simulink model "Drone_Simulation"  (R2020a)
settings: Solver=ode1  StartTime=0.0  StopTime=50  FixedStep=1e-3
values from neighbouring files (symbols this model uses):
  AeEMSC = 1    [Qball_X8_Model.m]
  alpha1TDDBSC = 1    [Qball_X8_Model.m]    (also in ReliabilityModel_Script.m = 0.7)
  bBNG = 1.2    [ReliabilityModel_Script.m]
  bEMSC = 1    [Qball_X8_Model.m]
  bEVCAP = 1    [Qball_X8_Model.m]    (also in ReliabilityModel_Script.m = 1.1)
  BNG_Motor1 = 0.8    [ReliabilityModel_Script.m]
  BNG_Motor2 = 1    [ReliabilityModel_Script.m]
  BNG_Motor3 = 1    [ReliabilityModel_Script.m]
  BNG_Motor4 = 1    [ReliabilityModel_Script.m]
  BNG_Motor5 = 1    [ReliabilityModel_Script.m]
  BNG_Motor6 = 1    [ReliabilityModel_Script.m]
  bp = 0.001    [ControlLawsScript.m]    (also in ControlLaws_Script.m)
  bq = 0.001    [ControlLawsScript.m]    (also in ControlLaws_Script.m)
  br = 0.001    [ControlLawsScript.m]    (also in ControlLaws_Script.m)
  bTDDBSC = 1    [Qball_X8_Model.m]    (also in ReliabilityModel_Script.m = 1.1)
  bWDG = 1    [Qball_X8_Model.m]    (also in ReliabilityModel_Script.m = 1.1)
  C_A = [     k_T           k_T          k_T                k_T          k_T         k_T ... (first row only)    [ControlLawsScript.m]    (also in ControlLaws_Script.m)
  C_mot = 1    [Qball_X8_Model.m]    (also in ReliabilityModel_Script.m = 17.46)
  C_th_esc = 1    [Qball_X8_Model.m]    (also in ReliabilityModel_Script.m = 1.67)
  CAPEV_Motor1 = 0.8    [ReliabilityModel_Script.m]
  CAPEV_Motor2 = 1    [ReliabilityModel_Script.m]
  CAPEV_Motor3 = 1    [ReliabilityModel_Script.m]
  CAPEV_Motor4 = 1    [ReliabilityModel_Script.m]
  CAPEV_Motor5 = 1    [ReliabilityModel_Script.m]
  CAPEV_Motor6 = 1    [ReliabilityModel_Script.m]
  cdx = cx*m    (= 17.4057414746)    [ControlLawsScript.m]    (also in ControlLaws_Script.m)
  cdy = cy*m    (= 17.4057414746)    [ControlLawsScript.m]    (also in ControlLaws_Script.m)
  cdz = cz*m    (= 17.4057414746)    [ControlLawsScript.m]    (also in ControlLaws_Script.m)
  EaEMSC = 1    [Qball_X8_Model.m]
  EaEVCAP = 1    [Qball_X8_Model.m]    (also in ReliabilityModel_Script.m = 0.94)
  EalphaTDDBSC = 1    [Qball_X8_Model.m]    (also in ReliabilityModel_Script.m = 0.7)
  EaTDDBSC = 1    [Qball_X8_Model.m]    (also in ReliabilityModel_Script.m = 0.7)
  EaWDG = 1    [Qball_X8_Model.m]    (also in ReliabilityModel_Script.m = 0.5)
  g = 9.80665    [ControlLawsScript.m]    (also in ControlLaws_Script.m; Qball_X8_Model.m = 9.87)
  JrefEMSC = 1    [Qball_X8_Model.m]
  Jz = 0.15887270137511    (= 0.158872701375)    [ControlLawsScript.m]    (also in ControlLaws_Script.m)
  k_b = 1    [Qball_X8_Model.m]    (also in ReliabilityModel_Script.m = -21.8546)
  Kp = (Jx/Tc)-bp    (= 4.11390529802)    [ControlLawsScript.m]    (also in ControlLaws_Script.m)
  Kp2 = Jx*((4/ts))*((-4/ts)+((bp+Kp)/Jx))/Kp    (= 6.72163348437)    [ControlLawsScript.m]    (also in ControlLaws_Script.m)
  Kq = (Jy/Tc)-bq    (= 4.12186008142)    [ControlLawsScript.m]    (also in ControlLaws_Script.m)
  Kq2 = Jy*((4/ts))*((-4/ts)+((bq+Kq)/Jy))/Kq    (= 6.72163033191)    [ControlLawsScript.m]    (also in ControlLaws_Script.m)
  Kr = (Jz/(tsy/25))-br    (= 7.94263506876)    [ControlLawsScript.m]    (also in ControlLaws_Script.m)
  Kr2 = Jz*((4/tsy))*((-4/tsy)+((br+Kr)/Jz))/Kr    (= 6.72084606682)    [ControlLawsScript.m]    (also in ControlLaws_Script.m)
  kv = 1/930    (= 0.0010752688172)    [StingerScript.m]
  Kx = abs(Kx)    [ControlLawsScript.m]    (also in ControlLaws_Script.m)
  Ky = abs(Ky)    [ControlLawsScript.m]    (also in ControlLaws_Script.m)
  Kz = (m/Tcz)-cz    (= 38.5143536865)    [ControlLawsScript.m]    (also in ControlLaws_Script.m)
  Kz2 = m*((4/tsz))*((-4/tsz)+((cz+Kz)/m))/Kz    (= 1.89810050529)    [ControlLawsScript.m]    (also in ControlLaws_Script.m)
  LnomEMSC = 1    [Qball_X8_Model.m]
  LnomEVCAP = 1    [Qball_X8_Model.m]    (also in ReliabilityModel_Script.m = 10800000)
  LnomTDDBSC = 1    [Qball_X8_Model.m]    (also in ReliabilityModel_Script.m = 9997200)
  LnomWDG = 1    [Qball_X8_Model.m]    (also in ReliabilityModel_Script.m = 72000000)
  m = 3.4811482949175    (= 3.48114829492)    [ControlLawsScript.m]    (also in ControlLaws_Script.m; Qball_X8_Model.m = 1.45)
  max_yaw_moment = k_y*hov_thrust/k_T    (= 0.323744079512)    [ControlLawsScript.m]    (also in ControlLaws_Script.m = 0.57666914163)
  NEMSC = 1    [Qball_X8_Model.m]
  nEVCAP = 1    [Qball_X8_Model.m]    (also in ReliabilityModel_Script.m)
  pconst = 2    [Qball_X8_Model.m]    (also in ReliabilityModel_Script.m)
  pitch_angle_limit = 32/R2D    (= 0.558505360638)    [ControlLawsScript.m]    (also in ControlLaws_Script.m)
  R2D = 180/pi    (= 57.2957795131)    [ControlLawsScript.m]    (also in ControlLaws_Script.m)
  R_th_esc = 1    [Qball_X8_Model.m]    (also in ReliabilityModel_Script.m = 5.14)
  R_th_mot = 1    [Qball_X8_Model.m]    (also in ReliabilityModel_Script.m = 8.59)
  Re = 0.008    [Qball_X8_Model.m]    (also in ReliabilityModel_Script.m)
  roll_angle_limit = 32/R2D    (= 0.558505360638)    [ControlLawsScript.m]    (also in ControlLaws_Script.m)
  RrefBNG = 0.9    [ReliabilityModel_Script.m]
  RrefEMSC = 1    [Qball_X8_Model.m]
  RrefEVCAP = 1    [Qball_X8_Model.m]    (also in ReliabilityModel_Script.m = 0.9)
  RrefTDDBSC = 1    [Qball_X8_Model.m]    (also in ReliabilityModel_Script.m = 0.37)
  RrefWDG = 1    [Qball_X8_Model.m]    (also in ReliabilityModel_Script.m = 0.98)
  SCTDDB_Motor1 = 0.8    [ReliabilityModel_Script.m]
  SCTDDB_Motor2 = 1    [ReliabilityModel_Script.m]
  SCTDDB_Motor3 = 1    [ReliabilityModel_Script.m]
  SCTDDB_Motor4 = 1    [ReliabilityModel_Script.m]
  SCTDDB_Motor5 = 1    [ReliabilityModel_Script.m]
  SCTDDB_Motor6 = 1    [ReliabilityModel_Script.m]
  T_amb = 1    [Qball_X8_Model.m]    (also in ReliabilityModel_Script.m = 20)
  T_amb_mot = 1    [Qball_X8_Model.m]    (also in ReliabilityModel_Script.m = 20)
  t_D_SCTDDB = 30    [ReliabilityModel_Script.m]
  TrefEMSC = 1    [Qball_X8_Model.m]
  TrefEVCAP = 1    [Qball_X8_Model.m]    (also in ReliabilityModel_Script.m = 105)
  TrefTDDBSC = 1    [Qball_X8_Model.m]    (also in ReliabilityModel_Script.m = 150)
  TrefWDG = 1    [Qball_X8_Model.m]    (also in ReliabilityModel_Script.m = 40)
  Ub = 12    [Qball_X8_Model.m]    (also in ReliabilityModel_Script.m)
  VmaxEVCAP = 1    [Qball_X8_Model.m]    (also in ReliabilityModel_Script.m = 35)
  VnomEVCAP = 1    [Qball_X8_Model.m]    (also in ReliabilityModel_Script.m = 35)
  WDG_Motor1 = 0.8    [ReliabilityModel_Script.m]
  WDG_Motor2 = 1    [ReliabilityModel_Script.m]
  WDG_Motor3 = 1    [ReliabilityModel_Script.m]
  WDG_Motor4 = 1    [ReliabilityModel_Script.m]
  WDG_Motor5 = 1    [ReliabilityModel_Script.m]
  WDG_Motor6 = 1    [ReliabilityModel_Script.m]
  z_x = cx    (= 5)    [ControlLawsScript.m]    (also in ControlLaws_Script.m)
  z_y = cy    (= 5)    [ControlLawsScript.m]    (also in ControlLaws_Script.m)
undefined symbols (not defined in the file or in its folder): FuselageContactForces, LeftAftArm, LeftAftSkid, LeftArm, LeftFrontArm, LeftFrontSkid, LeftSideContactForces, Lower, missionPlanX, missionPlanY, missionPlanYaw, missionPlanZ, Newton, Raphson, RightAftArm, RightAftSkid, RightArm, RightFrontArm, RightFrontSkid, RightSideContactForces, SkidsContactForces, timeConstant, Upper, X, Y, Z
libraries: sm_lib x90, nesl_utility x78, fl_lib x61, ee_lib x19, dspinverses x1, dspmtrx3 x1
(part 4 of 5)

== system Drone_Simulation/PLANT MODEL/ELECTRIC SYSTEM/Motor 4 ==
  Aerodynamic Drag : fl_lib/Mechanical/Mechanical Sources/Ideal Torque Source
  Controlled PWM Voltage : ee_lib/Integrated Circuits/Controlled PWM Voltage  F=freq Hz  TD=0 s  pulse_width_offset=0 s  pulse_min=0 s  Vmin=0 V  Vmax=5 V  Vm=1 V  pwm_or_av=1  event_type=2  sample_time=Samp_time s  u_min=0  u_max=1
      settings: InternalSimscapePortConfiguration="{\"Bottom\":[],\"Left\":[{\"id\":\"u\",\"label\":\"u\",\"type\":\"input\"}],\"Right\":[{\"id\":\"p2\",\"label\":\"PWM\",\"type\":\"foundation.electrical.electrical\"},{\"id\":\"n2\",\"label\":\"REF\",\"type\":\"foundation.electrical.electrical\"}],\"Top\":[]}"
  Current Sensor : fl_lib/Electrical/Electrical Sensors/Current Sensor
  DC Motor : ee_lib/Electromechanical/Brushed Motors/DC Motor  field_option=ee.enum.field_option.pm  Rf=100 Ohm  Lf=1 H  Laf=0.15 H  If0=0 A  parameterization=ee.enum.dcparam_option.circuit_param  Ra=R Ohm  La=100 uH  emf_or_torque=ee.enum.emf_or_torque.kv  Kv=Kv V/rpm  Ki=kv N*m/A  T_stall=0.1 N*m  w_max=4000 rpm  w_rated=2500 rpm  P_rated=10 W  V_rated=12 V  J=0 kg*m^2  lam_param=ee.enum.lam_param.current  lam=0.5e-5 N*m/(rad/s)  i_noload=Ic A  V_i_noload=14.8 V  speed0=0 rpm  alpha=3.93e-3 1/K  Tmeas=25 degC  thermal_mass=100 J/K  initial_temperature=25 degC
  H-Bridge : ee_lib/Semiconductors & Converters/Converters/H-Bridge  supply_ports=ee.enum.supply_ports.showsupply  Venable=0.01 V  Vmax=5 V  Vreverse=10000 V  Vbrake=10000 V  Vm=12 V  pwm_or_av=ee.enum.pwm_or_av.pwm  regenerative_braking_mode=ee.enum.converters.regenerative_braking_mode.always_enabled  discontinuous=ee.enum.current_profile.continuous  freewheeling_mode=ee.enum.converters.freewheeling_mode.two_switches_one_diode  Ron=0.00001 Ohm  Don=0.1 Ohm  Goff=1e-6 S  Rload=3.38+0.1 Ohm  Lload=1e-5 H  F=4 kHz  thermal_mass=100 J/K  initial_temperature=298.15 K  Ron2=0.1 Ohm  Don2=0.05 Ohm  Tmeas=298.15 K  Tmeas2=398.15 K
      settings: InternalSimscapePortConfiguration="{\"Bottom\":[],\"Left\":[{\"id\":\"ENA\",\"label\":\"PWM\",\"type\":\"foundation.electrical.electrical\"},{\"id\":\"REF\",\"label\":\"REF\",\"type\":\"foundation.electrical.electrical\"},{\"id\":\"REV\",\"label\":\"REV\",\"type\":\"foundation.electrical.electrical\"},{\"id\":\"BRK\",\"label\":\"BRK\",\"type\":\"foundation.electrical.electrical\"}],\"Right\":[{\"id\":\"p1\",\"label\":\"V+\",\"type\":\"foundation.electrical.electrical\"},{\"id\":\"p2\",\"label\":\"+\",\"type\":\"foundation.electrical.electrical\"},{\"id\":\"n2\",\"label\":\"-\",\"type\":\"foundation.electrical.electrical\"},{\"id\":\"n1\",\"label\":\"V-\",\"type\":\"foundation.electrical.electrical\"}],\"Top\":[]}"
  Ideal Rotational Motion Sensor : fl_lib/Mechanical/Mechanical Sensors/Ideal Rotational Motion Sensor  wrap_angle=simscape.enum.onoff.off  offset=0 deg
  Ideal Torque Sensor : fl_lib/Mechanical/Mechanical Sensors/Ideal Torque Sensor
  MRRef : fl_lib/Mechanical/Rotational Elements/Mechanical Rotational Reference
  Mechanical Rotational Reference2 : fl_lib/Mechanical/Rotational Elements/Mechanical Rotational Reference
  PS-Simulink : nesl_utility/PS-Simulink Converter  PhysicalDomain=network_engine_domain  SubClassName=ps_output  LeftPortType=input  RightPortType=output  PseudoPeriodic=off  Frequencies=[]  Unit=rpm  AffineConversion=off
  PS-Simulink Converter : nesl_utility/PS-Simulink Converter  PhysicalDomain=network_engine_domain  SubClassName=ps_output  LeftPortType=input  RightPortType=output  PseudoPeriodic=off  Frequencies=[]  Unit=inherit  AffineConversion=off
  PS-Simulink Converter1 : nesl_utility/PS-Simulink Converter  PhysicalDomain=network_engine_domain  SubClassName=ps_output  LeftPortType=input  RightPortType=output  PseudoPeriodic=off  Frequencies=[]  Unit=inherit  AffineConversion=off
  PS-Simulink Converter3 : nesl_utility/PS-Simulink Converter  PhysicalDomain=network_engine_domain  SubClassName=ps_output  LeftPortType=input  RightPortType=output  PseudoPeriodic=off  Frequencies=[]  Unit=inherit  AffineConversion=off
  PS-Simulink3 : nesl_utility/PS-Simulink Converter  PhysicalDomain=network_engine_domain  SubClassName=ps_output  LeftPortType=input  RightPortType=output  PseudoPeriodic=off  Frequencies=[]  Unit=A  AffineConversion=off
  Propeller Inertia : fl_lib/Mechanical/Rotational Elements/Inertia  inertia=J kg*m^2  w_specify=off  w_priority=High  w=0 rpm  w_nominal_specify=off  w_nominal_unit=rad/s  w_nominal_value=1  t_specify=off  t_priority=High  t=0 N*m  t_nominal_specify=off  t_nominal_unit=N*m  t_nominal_value=1
  RPM to Resistive Torque and Thrust : Subsystem
  Scope2 : Scope
  Signals : Subsystem
  Simulink-PS Converter : nesl_utility/Simulink-PS Converter  PhysicalDomain=network_engine_domain  SubClassName=ps_input  LeftPortType=input  RightPortType=output  PseudoPeriodic=off  Frequencies=[]  NoiseDistribution=none  NoiseParameters=[]  Unit=1  AffineConversion=off  FilteringAndDerivatives=filter  SimscapeFilterOrder=1  InputFilterTimeConstant=0.001  UdotUserProvided=0
  Simulink-PS Converter1 : nesl_utility/Simulink-PS Converter  PhysicalDomain=network_engine_domain  SubClassName=ps_input  LeftPortType=input  RightPortType=output  PseudoPeriodic=off  Frequencies=[]  NoiseDistribution=none  NoiseParameters=[]  Unit=N*m  AffineConversion=off  FilteringAndDerivatives=provide  SimscapeFilterOrder=1  InputFilterTimeConstant=0.001  UdotUserProvided=0
  Sum : Sum  Inputs=|+-
  Terminator : Terminator
  Transfer Fcn2 : TransferFcn  Numerator=[1*2*pi]  Denominator=[1 1*2*pi]
  Transfer Fcn3 : TransferFcn  Numerator=[1*2*pi]  Denominator=[1 1*2*pi]
  Visualization : Scope  NumInputPorts=4
  Voltage Sensor1 : fl_lib/Electrical/Electrical Sensors/Voltage Sensor
  Connection Port1 : PMIOPort  Side=Left
  Connection Port : PMIOPort  Port=2  Side=Right
  tag scope: AngleMotor4=global, AngularSpeed4=global, I_ESC_OUT4=global, Thrust4=global, Trq4=global, V_ESC_OUT4=global
  wires:
  RPM to Resistive Torque and Thrust/2(Resistive Torque) -> [Trq4], Simulink-PS Converter1/1  "Torque"
  [AngularSpeed4] -> RPM to Resistive Torque and Thrust/1(Angular Speed)
  RPM to Resistive Torque and Thrust/1(Thrust) -> [Thrust4]  "Thrust"
  PS-Simulink Converter1/1 -> Terminator/1
  PS-Simulink/1 -> Scope2/1, Sum/2, [AngularSpeed4]  "Motor RPM"
  [ReqSpeedMotor4] -> Sum/1  "Motor Desired Speed"
  Transfer Fcn2/1 -> [I_ESC_OUT4]
  PS-Simulink3/1 -> Transfer Fcn2/1  "Motor Current"
  PS-Simulink Converter3/1 -> Transfer Fcn3/1  "Motor Voltage"
  Transfer Fcn3/1 -> [V_ESC_OUT4]
  PS-Simulink Converter/1 -> [AngleMotor4]
  Sum/1 -> Simulink-PS Converter/1
  Signals/4(V) -> Visualization/4
  Signals/3(Trq) -> Visualization/3
  Signals/2(ia) -> Visualization/2
  Signals/1(Spd) -> Visualization/1
  connections:
  Ideal Rotational Motion Sensor/RConn2 -- PS-Simulink/LConn1
  PS-Simulink Converter1/LConn1 -- Ideal Torque Sensor/RConn2
  Ideal Torque Sensor/RConn1 -- Aerodynamic Drag/LConn1
  Simulink-PS Converter1/RConn1 -- Aerodynamic Drag/RConn1
  Mechanical Rotational Reference2/LConn1 -- Aerodynamic Drag/RConn2
  Ideal Torque Sensor/LConn1 -- DC Motor/LConn2 -- Propeller Inertia/LConn1 -- Ideal Rotational Motion Sensor/LConn1
  Ideal Rotational Motion Sensor/RConn1 -- MRRef/LConn1 -- DC Motor/RConn2
  H-Bridge/RConn4 -- Connection Port/RConn1 -- H-Bridge/LConn3 -- Controlled PWM Voltage/RConn2 -- H-Bridge/LConn2 -- H-Bridge/LConn4
  Controlled PWM Voltage/RConn1 -- H-Bridge/LConn1
  Simulink-PS Converter/RConn1 -- Controlled PWM Voltage/LConn1
  H-Bridge/RConn3 -- Voltage Sensor1/RConn2 -- DC Motor/RConn1
  Connection Port1/RConn1 -- H-Bridge/RConn1
  Current Sensor/LConn1 -- Voltage Sensor1/LConn1 -- H-Bridge/RConn2
  PS-Simulink3/LConn1 -- Current Sensor/RConn1
  Current Sensor/RConn2 -- DC Motor/LConn1
  Voltage Sensor1/RConn1 -- PS-Simulink Converter3/LConn1
  PS-Simulink Converter/LConn1 -- Ideal Rotational Motion Sensor/RConn3

== system Drone_Simulation/PLANT MODEL/ELECTRIC SYSTEM/Motor 5 ==
  Aerodynamic Drag : fl_lib/Mechanical/Mechanical Sources/Ideal Torque Source
  Controlled PWM Voltage : ee_lib/Integrated Circuits/Controlled PWM Voltage  F=freq Hz  TD=0 s  pulse_width_offset=0 s  pulse_min=0 s  Vmin=0 V  Vmax=5 V  Vm=1 V  pwm_or_av=1  event_type=2  sample_time=Samp_time s  u_min=0  u_max=1
      settings: InternalSimscapePortConfiguration="{\"Bottom\":[],\"Left\":[{\"id\":\"u\",\"label\":\"u\",\"type\":\"input\"}],\"Right\":[{\"id\":\"p2\",\"label\":\"PWM\",\"type\":\"foundation.electrical.electrical\"},{\"id\":\"n2\",\"label\":\"REF\",\"type\":\"foundation.electrical.electrical\"}],\"Top\":[]}"
  Current Sensor : fl_lib/Electrical/Electrical Sensors/Current Sensor
  DC Motor : ee_lib/Electromechanical/Brushed Motors/DC Motor  field_option=ee.enum.field_option.pm  Rf=100 Ohm  Lf=1 H  Laf=0.15 H  If0=0 A  parameterization=ee.enum.dcparam_option.circuit_param  Ra=R Ohm  La=100 uH  emf_or_torque=ee.enum.emf_or_torque.kv  Kv=Kv V/rpm  Ki=kv N*m/A  T_stall=0.1 N*m  w_max=4000 rpm  w_rated=2500 rpm  P_rated=10 W  V_rated=12 V  J=0 kg*m^2  lam_param=ee.enum.lam_param.current  lam=0.5e-5 N*m/(rad/s)  i_noload=Ic A  V_i_noload=14.8 V  speed0=0 rpm  alpha=3.93e-3 1/K  Tmeas=25 degC  thermal_mass=100 J/K  initial_temperature=25 degC
  H-Bridge : ee_lib/Semiconductors & Converters/Converters/H-Bridge  supply_ports=ee.enum.supply_ports.showsupply  Venable=0.01 V  Vmax=5 V  Vreverse=10000 V  Vbrake=10000 V  Vm=12 V  pwm_or_av=ee.enum.pwm_or_av.pwm  regenerative_braking_mode=ee.enum.converters.regenerative_braking_mode.always_enabled  discontinuous=ee.enum.current_profile.continuous  freewheeling_mode=ee.enum.converters.freewheeling_mode.two_switches_one_diode  Ron=0.00001 Ohm  Don=0.1 Ohm  Goff=1e-6 S  Rload=3.38+0.1 Ohm  Lload=1e-5 H  F=4 kHz  thermal_mass=100 J/K  initial_temperature=298.15 K  Ron2=0.1 Ohm  Don2=0.05 Ohm  Tmeas=298.15 K  Tmeas2=398.15 K
      settings: InternalSimscapePortConfiguration="{\"Bottom\":[],\"Left\":[{\"id\":\"ENA\",\"label\":\"PWM\",\"type\":\"foundation.electrical.electrical\"},{\"id\":\"REF\",\"label\":\"REF\",\"type\":\"foundation.electrical.electrical\"},{\"id\":\"REV\",\"label\":\"REV\",\"type\":\"foundation.electrical.electrical\"},{\"id\":\"BRK\",\"label\":\"BRK\",\"type\":\"foundation.electrical.electrical\"}],\"Right\":[{\"id\":\"p1\",\"label\":\"V+\",\"type\":\"foundation.electrical.electrical\"},{\"id\":\"p2\",\"label\":\"+\",\"type\":\"foundation.electrical.electrical\"},{\"id\":\"n2\",\"label\":\"-\",\"type\":\"foundation.electrical.electrical\"},{\"id\":\"n1\",\"label\":\"V-\",\"type\":\"foundation.electrical.electrical\"}],\"Top\":[]}"
  Ideal Rotational Motion Sensor : fl_lib/Mechanical/Mechanical Sensors/Ideal Rotational Motion Sensor  wrap_angle=simscape.enum.onoff.off  offset=0 deg
  Ideal Torque Sensor : fl_lib/Mechanical/Mechanical Sensors/Ideal Torque Sensor
  MRRef : fl_lib/Mechanical/Rotational Elements/Mechanical Rotational Reference
  Mechanical Rotational Reference2 : fl_lib/Mechanical/Rotational Elements/Mechanical Rotational Reference
  PS-Simulink : nesl_utility/PS-Simulink Converter  PhysicalDomain=network_engine_domain  SubClassName=ps_output  LeftPortType=input  RightPortType=output  PseudoPeriodic=off  Frequencies=[]  Unit=rpm  AffineConversion=off
  PS-Simulink Converter : nesl_utility/PS-Simulink Converter  PhysicalDomain=network_engine_domain  SubClassName=ps_output  LeftPortType=input  RightPortType=output  PseudoPeriodic=off  Frequencies=[]  Unit=inherit  AffineConversion=off
  PS-Simulink Converter1 : nesl_utility/PS-Simulink Converter  PhysicalDomain=network_engine_domain  SubClassName=ps_output  LeftPortType=input  RightPortType=output  PseudoPeriodic=off  Frequencies=[]  Unit=inherit  AffineConversion=off
  PS-Simulink Converter3 : nesl_utility/PS-Simulink Converter  PhysicalDomain=network_engine_domain  SubClassName=ps_output  LeftPortType=input  RightPortType=output  PseudoPeriodic=off  Frequencies=[]  Unit=inherit  AffineConversion=off
  PS-Simulink3 : nesl_utility/PS-Simulink Converter  PhysicalDomain=network_engine_domain  SubClassName=ps_output  LeftPortType=input  RightPortType=output  PseudoPeriodic=off  Frequencies=[]  Unit=A  AffineConversion=off
  Propeller Inertia : fl_lib/Mechanical/Rotational Elements/Inertia  inertia=J kg*m^2  w_specify=off  w_priority=High  w=0 rpm  w_nominal_specify=off  w_nominal_unit=rad/s  w_nominal_value=1  t_specify=off  t_priority=High  t=0 N*m  t_nominal_specify=off  t_nominal_unit=N*m  t_nominal_value=1
  RPM to Resistive Torque and Thrust : Subsystem
  Scope3 : Scope
  Signals : Subsystem
  Simulink-PS Converter : nesl_utility/Simulink-PS Converter  PhysicalDomain=network_engine_domain  SubClassName=ps_input  LeftPortType=input  RightPortType=output  PseudoPeriodic=off  Frequencies=[]  NoiseDistribution=none  NoiseParameters=[]  Unit=1  AffineConversion=off  FilteringAndDerivatives=filter  SimscapeFilterOrder=1  InputFilterTimeConstant=0.001  UdotUserProvided=0
  Simulink-PS Converter1 : nesl_utility/Simulink-PS Converter  PhysicalDomain=network_engine_domain  SubClassName=ps_input  LeftPortType=input  RightPortType=output  PseudoPeriodic=off  Frequencies=[]  NoiseDistribution=none  NoiseParameters=[]  Unit=N*m  AffineConversion=off  FilteringAndDerivatives=provide  SimscapeFilterOrder=1  InputFilterTimeConstant=0.001  UdotUserProvided=0
  Sum : Sum  Inputs=|+-
  Terminator : Terminator
  Transfer Fcn2 : TransferFcn  Numerator=[1*2*pi]  Denominator=[1 1*2*pi]
  Transfer Fcn3 : TransferFcn  Numerator=[1*2*pi]  Denominator=[1 1*2*pi]
  Visualization : Scope  NumInputPorts=4
  Voltage Sensor1 : fl_lib/Electrical/Electrical Sensors/Voltage Sensor
  Connection Port1 : PMIOPort  Side=Left
  Connection Port : PMIOPort  Port=2  Side=Right
  tag scope: AngleMotor5=global, AngularSpeed5=global, I_ESC_OUT5=global, Thrust5=global, Trq5=global, V_ESC_OUT5=global
  wires:
  RPM to Resistive Torque and Thrust/2(Resistive Torque) -> [Trq5], Simulink-PS Converter1/1  "Torque"
  [AngularSpeed5] -> RPM to Resistive Torque and Thrust/1(Angular Speed)
  RPM to Resistive Torque and Thrust/1(Thrust) -> [Thrust5]  "Thrust"
  PS-Simulink Converter1/1 -> Terminator/1
  PS-Simulink/1 -> Scope3/1, Sum/2, [AngularSpeed5]  "Motor RPM"
  [ReqSpeedMotor5] -> Sum/1  "Motor Desired Speed"
  PS-Simulink3/1 -> Transfer Fcn2/1  "Motor Current"
  Transfer Fcn2/1 -> [I_ESC_OUT5]
  PS-Simulink Converter3/1 -> Transfer Fcn3/1  "Motor Voltage"
  Transfer Fcn3/1 -> [V_ESC_OUT5]
  PS-Simulink Converter/1 -> [AngleMotor5]
  Sum/1 -> Simulink-PS Converter/1
  Signals/4(V) -> Visualization/4
  Signals/3(Trq) -> Visualization/3
  Signals/2(ia) -> Visualization/2
  Signals/1(Spd) -> Visualization/1
  connections:
  Ideal Rotational Motion Sensor/RConn2 -- PS-Simulink/LConn1
  PS-Simulink Converter1/LConn1 -- Ideal Torque Sensor/RConn2
  Ideal Torque Sensor/RConn1 -- Aerodynamic Drag/LConn1
  Simulink-PS Converter1/RConn1 -- Aerodynamic Drag/RConn1
  Mechanical Rotational Reference2/LConn1 -- Aerodynamic Drag/RConn2
  Ideal Torque Sensor/LConn1 -- DC Motor/LConn2 -- Propeller Inertia/LConn1 -- Ideal Rotational Motion Sensor/LConn1
  Ideal Rotational Motion Sensor/RConn1 -- MRRef/LConn1 -- DC Motor/RConn2
  Connection Port/RConn1 -- H-Bridge/RConn4 -- H-Bridge/LConn3 -- Controlled PWM Voltage/RConn2 -- H-Bridge/LConn2 -- H-Bridge/LConn4
  H-Bridge/RConn2 -- Voltage Sensor1/LConn1 -- Current Sensor/LConn1
  Controlled PWM Voltage/RConn1 -- H-Bridge/LConn1
  Simulink-PS Converter/RConn1 -- Controlled PWM Voltage/LConn1
  H-Bridge/RConn3 -- DC Motor/RConn1 -- Voltage Sensor1/RConn2
  Connection Port1/RConn1 -- H-Bridge/RConn1
  PS-Simulink3/LConn1 -- Current Sensor/RConn1
  Current Sensor/RConn2 -- DC Motor/LConn1
  Voltage Sensor1/RConn1 -- PS-Simulink Converter3/LConn1
  PS-Simulink Converter/LConn1 -- Ideal Rotational Motion Sensor/RConn3

== system Drone_Simulation/PLANT MODEL/ELECTRIC SYSTEM/Motor 6 ==
  Aerodynamic Drag : fl_lib/Mechanical/Mechanical Sources/Ideal Torque Source
  Controlled PWM Voltage : ee_lib/Integrated Circuits/Controlled PWM Voltage  F=freq Hz  TD=0 s  pulse_width_offset=0 s  pulse_min=0 s  Vmin=0 V  Vmax=5 V  Vm=1 V  pwm_or_av=1  event_type=2  sample_time=Samp_time s  u_min=0  u_max=1
      settings: InternalSimscapePortConfiguration="{\"Bottom\":[],\"Left\":[{\"id\":\"u\",\"label\":\"u\",\"type\":\"input\"}],\"Right\":[{\"id\":\"p2\",\"label\":\"PWM\",\"type\":\"foundation.electrical.electrical\"},{\"id\":\"n2\",\"label\":\"REF\",\"type\":\"foundation.electrical.electrical\"}],\"Top\":[]}"
  Current Sensor : fl_lib/Electrical/Electrical Sensors/Current Sensor
  DC Motor : ee_lib/Electromechanical/Brushed Motors/DC Motor  field_option=ee.enum.field_option.pm  Rf=100 Ohm  Lf=1 H  Laf=0.15 H  If0=0 A  parameterization=ee.enum.dcparam_option.circuit_param  Ra=R Ohm  La=100 uH  emf_or_torque=ee.enum.emf_or_torque.kv  Kv=Kv V/rpm  Ki=kv N*m/A  T_stall=0.1 N*m  w_max=4000 rpm  w_rated=2500 rpm  P_rated=10 W  V_rated=12 V  J=0 kg*m^2  lam_param=ee.enum.lam_param.current  lam=0.5e-5 N*m/(rad/s)  i_noload=Ic A  V_i_noload=14.8 V  speed0=0 rpm  alpha=3.93e-3 1/K  Tmeas=25 degC  thermal_mass=100 J/K  initial_temperature=25 degC
  H-Bridge : ee_lib/Semiconductors & Converters/Converters/H-Bridge  supply_ports=ee.enum.supply_ports.showsupply  Venable=0.01 V  Vmax=5 V  Vreverse=10000 V  Vbrake=10000 V  Vm=12 V  pwm_or_av=ee.enum.pwm_or_av.pwm  regenerative_braking_mode=ee.enum.converters.regenerative_braking_mode.always_enabled  discontinuous=ee.enum.current_profile.continuous  freewheeling_mode=ee.enum.converters.freewheeling_mode.two_switches_one_diode  Ron=0.00001 Ohm  Don=0.1 Ohm  Goff=1e-6 S  Rload=3.38+0.1 Ohm  Lload=1e-5 H  F=4 kHz  thermal_mass=100 J/K  initial_temperature=298.15 K  Ron2=0.1 Ohm  Don2=0.05 Ohm  Tmeas=298.15 K  Tmeas2=398.15 K
      settings: InternalSimscapePortConfiguration="{\"Bottom\":[],\"Left\":[{\"id\":\"ENA\",\"label\":\"PWM\",\"type\":\"foundation.electrical.electrical\"},{\"id\":\"REF\",\"label\":\"REF\",\"type\":\"foundation.electrical.electrical\"},{\"id\":\"REV\",\"label\":\"REV\",\"type\":\"foundation.electrical.electrical\"},{\"id\":\"BRK\",\"label\":\"BRK\",\"type\":\"foundation.electrical.electrical\"}],\"Right\":[{\"id\":\"p1\",\"label\":\"V+\",\"type\":\"foundation.electrical.electrical\"},{\"id\":\"p2\",\"label\":\"+\",\"type\":\"foundation.electrical.electrical\"},{\"id\":\"n2\",\"label\":\"-\",\"type\":\"foundation.electrical.electrical\"},{\"id\":\"n1\",\"label\":\"V-\",\"type\":\"foundation.electrical.electrical\"}],\"Top\":[]}"
  Ideal Rotational Motion Sensor : fl_lib/Mechanical/Mechanical Sensors/Ideal Rotational Motion Sensor  wrap_angle=simscape.enum.onoff.off  offset=0 deg
  Ideal Torque Sensor : fl_lib/Mechanical/Mechanical Sensors/Ideal Torque Sensor
  MRRef : fl_lib/Mechanical/Rotational Elements/Mechanical Rotational Reference
  Mechanical Rotational Reference2 : fl_lib/Mechanical/Rotational Elements/Mechanical Rotational Reference
  PS-Simulink : nesl_utility/PS-Simulink Converter  PhysicalDomain=network_engine_domain  SubClassName=ps_output  LeftPortType=input  RightPortType=output  PseudoPeriodic=off  Frequencies=[]  Unit=rpm  AffineConversion=off
  PS-Simulink Converter : nesl_utility/PS-Simulink Converter  PhysicalDomain=network_engine_domain  SubClassName=ps_output  LeftPortType=input  RightPortType=output  PseudoPeriodic=off  Frequencies=[]  Unit=inherit  AffineConversion=off
  PS-Simulink Converter1 : nesl_utility/PS-Simulink Converter  PhysicalDomain=network_engine_domain  SubClassName=ps_output  LeftPortType=input  RightPortType=output  PseudoPeriodic=off  Frequencies=[]  Unit=inherit  AffineConversion=off
  PS-Simulink Converter3 : nesl_utility/PS-Simulink Converter  PhysicalDomain=network_engine_domain  SubClassName=ps_output  LeftPortType=input  RightPortType=output  PseudoPeriodic=off  Frequencies=[]  Unit=inherit  AffineConversion=off
  PS-Simulink3 : nesl_utility/PS-Simulink Converter  PhysicalDomain=network_engine_domain  SubClassName=ps_output  LeftPortType=input  RightPortType=output  PseudoPeriodic=off  Frequencies=[]  Unit=A  AffineConversion=off
  Propeller Inertia : fl_lib/Mechanical/Rotational Elements/Inertia  inertia=J kg*m^2  w_specify=off  w_priority=High  w=0 rpm  w_nominal_specify=off  w_nominal_unit=rad/s  w_nominal_value=1  t_specify=off  t_priority=High  t=0 N*m  t_nominal_specify=off  t_nominal_unit=N*m  t_nominal_value=1
  RPM to Resistive Torque and Thrust : Subsystem
  Signals : Subsystem
  Simulink-PS Converter : nesl_utility/Simulink-PS Converter  PhysicalDomain=network_engine_domain  SubClassName=ps_input  LeftPortType=input  RightPortType=output  PseudoPeriodic=off  Frequencies=[]  NoiseDistribution=none  NoiseParameters=[]  Unit=1  AffineConversion=off  FilteringAndDerivatives=filter  SimscapeFilterOrder=1  InputFilterTimeConstant=0.001  UdotUserProvided=0
  Simulink-PS Converter1 : nesl_utility/Simulink-PS Converter  PhysicalDomain=network_engine_domain  SubClassName=ps_input  LeftPortType=input  RightPortType=output  PseudoPeriodic=off  Frequencies=[]  NoiseDistribution=none  NoiseParameters=[]  Unit=N*m  AffineConversion=off  FilteringAndDerivatives=provide  SimscapeFilterOrder=1  InputFilterTimeConstant=0.001  UdotUserProvided=0
  Sum : Sum  Inputs=|+-
  Terminator : Terminator
  Transfer Fcn2 : TransferFcn  Numerator=[1*2*pi]  Denominator=[1 1*2*pi]
  Transfer Fcn3 : TransferFcn  Numerator=[1*2*pi]  Denominator=[1 1*2*pi]
  Visualization : Scope  NumInputPorts=4
  Voltage Sensor1 : fl_lib/Electrical/Electrical Sensors/Voltage Sensor
  Connection Port1 : PMIOPort  Side=Left
  Connection Port : PMIOPort  Port=2  Side=Right
  tag scope: AngleMotor6=global, AngularSpeed6=global, I_ESC_OUT6=global, Thrust6=global, Trq6=global, V_ESC_OUT6=global
  wires:
  RPM to Resistive Torque and Thrust/2(Resistive Torque) -> [Trq6], Simulink-PS Converter1/1  "Torque"
  [AngularSpeed6] -> RPM to Resistive Torque and Thrust/1(Angular Speed)
  RPM to Resistive Torque and Thrust/1(Thrust) -> [Thrust6]  "Thrust"
  PS-Simulink Converter1/1 -> Terminator/1
  PS-Simulink/1 -> Sum/2, [AngularSpeed6]  "Motor RPM"
  [ReqSpeedMotor6] -> Sum/1  "Motor Desired Speed"
  PS-Simulink3/1 -> Transfer Fcn2/1  "Motor Current"
  Transfer Fcn2/1 -> [I_ESC_OUT6]
  Transfer Fcn3/1 -> [V_ESC_OUT6]
  PS-Simulink Converter3/1 -> Transfer Fcn3/1  "Motor Voltage"
  PS-Simulink Converter/1 -> [AngleMotor6]
  Sum/1 -> Simulink-PS Converter/1
  Signals/3(Trq) -> Visualization/3
  Signals/1(Spd) -> Visualization/1
  Signals/4(V) -> Visualization/4
  Signals/2(ia) -> Visualization/2
  connections:
  Ideal Rotational Motion Sensor/RConn2 -- PS-Simulink/LConn1
  PS-Simulink Converter1/LConn1 -- Ideal Torque Sensor/RConn2
  Ideal Torque Sensor/RConn1 -- Aerodynamic Drag/LConn1
  Simulink-PS Converter1/RConn1 -- Aerodynamic Drag/RConn1
  Mechanical Rotational Reference2/LConn1 -- Aerodynamic Drag/RConn2
  Ideal Torque Sensor/LConn1 -- DC Motor/LConn2 -- Propeller Inertia/LConn1 -- Ideal Rotational Motion Sensor/LConn1
  Ideal Rotational Motion Sensor/RConn1 -- MRRef/LConn1 -- DC Motor/RConn2
  H-Bridge/RConn4 -- H-Bridge/LConn3 -- Controlled PWM Voltage/RConn2 -- H-Bridge/LConn2 -- H-Bridge/LConn4 -- Connection Port/RConn1
  H-Bridge/RConn2 -- Voltage Sensor1/LConn1 -- Current Sensor/LConn1
  Controlled PWM Voltage/RConn1 -- H-Bridge/LConn1
  Controlled PWM Voltage/LConn1 -- Simulink-PS Converter/RConn1
  DC Motor/RConn1 -- H-Bridge/RConn3 -- Voltage Sensor1/RConn2
  Connection Port1/RConn1 -- H-Bridge/RConn1
  PS-Simulink3/LConn1 -- Current Sensor/RConn1
  Current Sensor/RConn2 -- DC Motor/LConn1
  Voltage Sensor1/RConn1 -- PS-Simulink Converter3/LConn1
  PS-Simulink Converter/LConn1 -- Ideal Rotational Motion Sensor/RConn3

== system Drone_Simulation/PLANT MODEL/ELECTRIC SYSTEM/Subsystem ==
  In1 : Inport
  1-D Lookup Table : Lookup_n-D  NumberOfTableDimensions=1  BreakpointsForDimension1=[0,0.05,0.1,0.15,0.2,0.25,0.3,0.35,0.4,0.45,0.5,0.55,0.6,0.65,0.7,0.75,0.8,0.85,0.9,0.95,1]  Table=[0,12,13,13.4,13.62,13.75,13.85,13.91,13.95,14,14,14,14,14,14,14,14,14,14,14.8,16.8]  InternalRulePriority=Speed  RndMeth=Simplest  InputSameDT=on
  Battery Capacity : Constant  Value=18720
  Current Sign Saturation : Saturate  UpperLimit=350  LowerLimit=0
  Current integration : Integrator
  SOC Fraction : Product  Inputs=/*
  Scope1 : Scope
  Simulink-PS Converter : nesl_utility/Simulink-PS Converter  PhysicalDomain=network_engine_domain  SubClassName=ps_input  LeftPortType=input  RightPortType=output  PseudoPeriodic=off  Frequencies=[]  NoiseDistribution=none  NoiseParameters=[]  Unit=V  AffineConversion=off  FilteringAndDerivatives=filter  SimscapeFilterOrder=1  InputFilterTimeConstant=0.001  UdotUserProvided=0
  Sum : Sum  Inputs=+|-
  output : PMIOPort  Side=Right
  wires:
  Battery Capacity/1 -> SOC Fraction/1, Sum/1
  1-D Lookup Table/1 -> Simulink-PS Converter/1
  In1/1 -> Scope1/1, Current Sign Saturation/1
  SOC Fraction/1 -> 1-D Lookup Table/1
  Current Sign Saturation/1 -> Current integration/1
  Sum/1 -> SOC Fraction/2
  Current integration/1 -> Sum/2
  connections:
  Simulink-PS Converter/RConn1 -- output/RConn1

== system Drone_Simulation/PLANT MODEL/ELECTRIC SYSTEM/Subsystem1 ==
  In1 : Inport
  1-D Lookup Table : Lookup_n-D  NumberOfTableDimensions=1  BreakpointsForDimension1=[0,0.05,0.1,0.15,0.2,0.25,0.3,0.35,0.4,0.45,0.5,0.55,0.6,0.65,0.7,0.75,0.8,0.85,0.9,0.95,1]  Table=[0,12,13,13.4,13.62,13.75,13.85,13.91,13.95,14,14,14,14,14,14,14,14,14,14,14.8,16.8]  InternalRulePriority=Speed  RndMeth=Simplest  InputSameDT=on
  Battery Capacity : Constant  Value=18720
  Current Sign Saturation : Saturate  UpperLimit=350  LowerLimit=0
  Current integration : Integrator
  SOC Fraction : Product  Inputs=/*
  Scope1 : Scope
  Simulink-PS Converter : nesl_utility/Simulink-PS Converter  PhysicalDomain=network_engine_domain  SubClassName=ps_input  LeftPortType=input  RightPortType=output  PseudoPeriodic=off  Frequencies=[]  NoiseDistribution=none  NoiseParameters=[]  Unit=V  AffineConversion=off  FilteringAndDerivatives=filter  SimscapeFilterOrder=1  InputFilterTimeConstant=0.001  UdotUserProvided=0
  Sum : Sum  Inputs=+|-
  output : PMIOPort  Side=Right
  wires:
  Battery Capacity/1 -> SOC Fraction/1, Sum/1
  1-D Lookup Table/1 -> Simulink-PS Converter/1
  In1/1 -> Scope1/1, Current Sign Saturation/1
  SOC Fraction/1 -> 1-D Lookup Table/1
  Current Sign Saturation/1 -> Current integration/1
  Sum/1 -> SOC Fraction/2
  Current integration/1 -> Sum/2
  connections:
  Simulink-PS Converter/RConn1 -- output/RConn1

== system Drone_Simulation/PLANT MODEL/ENVIRONMENT/Ground ==
  Displacement : sm_lib/Frames and Transforms/Rigid Transform  TranslationMethod=StandardAxis  TranslationStandardOffset=P/2+Z+0.01  TranslationLengthUnit=m  TranslationStandardAxis=+Z  TranslationCartesianOffset=[0 0 0]  TranslationROffset=0  TranslationROffsetUnits=m  TranslationZOffset=0  TranslationZOffsetUnits=m  TranslationThetaOffset=0  TranslationThetaOffsetUnits=deg  RotationMethod=None  RotationAngleUnits=deg  RotationStandardAxis=+X  RotationAngle=90  RotationArbitraryAxis=[0 0 1]  FollAlignAxisA=+X  BaseAlignAxisA=+Y  FollAlignAxisB=+Y  BaseAlignAxisB=+Z  RotationSequenceAxes=FollowerAxes  RotationSequence=XYX  RotationSequenceAngles=[0 0 0]  RotationSequenceAnglesUnits=deg  RotationMatrix=[1 0 0; 0 1 0; 0 0 1]
  Earth : sm_lib/Body Elements/Brick Solid  GraphicAmbientColor=[0.15 0.15 0.15 1.0]  BasedOnType=Density  BrickDimensions=[E E P]  BrickDimensionUnits=m  CenterOfMass=[0 0 0]  CenterOfMassUnits=m  GraphicDiffuseColor=rgbE  Density=rhoE  DensityUnits=kg/m^3  DoExposeReferenceFrame=on  GraphicEmissiveColor=[0.0 0.0 0.0 1.0]  ExportEntireGeometry=on  SerializedFrames=<Frames/>  MarkerShape=Sphere  MarkerSize=10  GraphicType=FromGeometry  InertiaType=CalculateFromGeometry  Mass=1  MassUnits=kg  MomentsOfInertia=[1 1 1]  MomentsOfInertiaUnits=kg*m^2  GraphicOpacity=opE  ProductsOfInertia=[0 0 0]  ProductsOfInertiaUnits=kg*m^2  GraphicShininess=75  GraphicSpecularColor=[0.5 0.5 0.5 1.0]  GraphicVisPropType=SimpleVisualProperties
  Launch Insignia : sm_lib/Body Elements/Extruded Solid  GraphicAmbientColor=[0.15 0.15 0.15 1.0]  BasedOnType=Density  CenterOfMass=[0 0 0]  CenterOfMassUnits=m  GraphicDiffuseColor=[1.0 0.2 0.2]  ExportConvexHullGeometry=off  ExtrusionCrossSection=[0.15 0.15; -0.15 0.15; -0.15 0.75; -0.6 0.75; -0.6 -0.75; -0.15 -0.75; -0.15 -0.15; 0.15 -0.15; 0.15 -0.75; 0.6 -0.75; 0.6 0.75; 0.15 0.75]*0.5  ExtrusionCrossSectionUnits=m  Density=1  DensityUnits=kg/m^3  DoExposeReferenceFrame=on  GraphicEmissiveColor=[0.0 0.0 0.0 1.0]  ExportEntireGeometry=off  ExtrusionLength=0.002  ExtrusionLengthUnits=m  ExtrusionType=General  SerializedFrames=<Frames/>  MarkerShape=Sphere  MarkerSize=10  GraphicType=FromGeometry  InertiaType=CalculateFromGeometry  Mass=1  MassUnits=kg  MomentsOfInertia=[1 1 1]  MomentsOfInertiaUnits=kg*m^2  PolygonNumSides=3  GraphicOpacity=1.0  PolygonOuterRadius=1  PolygonOuterRadiusUnits=m  ProductsOfInertia=[0 0 0]  ProductsOfInertiaUnits=kg*m^2  GraphicShininess=75  GraphicSpecularColor=[0.5 0.5 0.5 1.0]  GraphicVisPropType=SimpleVisualProperties
  Launch Ring : sm_lib/Body Elements/Revolved Solid  GraphicAmbientColor=[0.15 0.15 0.15 1.0]  BasedOnType=Density  CenterOfMass=[0 0 0]  CenterOfMassUnits=m  GraphicDiffuseColor=[0.0 0.2 0.8]  ExportConvexHullGeometry=off  Density=1000  DensityUnits=kg/m^3  DoExposeReferenceFrame=on  GraphicEmissiveColor=[0.0 0.0 0.0 1.0]  ExportEntireGeometry=off  SerializedFrames=<Frames/>  MarkerShape=Sphere  MarkerSize=10  GraphicType=FromGeometry  InertiaType=CalculateFromGeometry  Mass=1  MassUnits=kg  MomentsOfInertia=[1 1 1]  MomentsOfInertiaUnits=kg*m^2  GraphicOpacity=1.0  ProductsOfInertia=[0 0 0]  ProductsOfInertiaUnits=kg*m^2  RevolutionCrossSection=[0.5 0.001; 0.5 -0.001; 0.75 -0.001; 0.75 0.001]  RevolutionCrossSectionUnits=m  RevolutionAngle=180  RevolutionAngleUnits=deg  RevolutionExtent=Full  GraphicShininess=75  GraphicSpecularColor=[0.5 0.5 0.5 1.0]  GraphicVisPropType=SimpleVisualProperties
  Transform Launch : sm_lib/Frames and Transforms/Rigid Transform  TranslationMethod=StandardAxis  TranslationStandardOffset=P/2+Z-0.3  TranslationLengthUnit=m  TranslationStandardAxis=+Z  TranslationCartesianOffset=P/2+Z+0.01  TranslationROffset=0  TranslationROffsetUnits=m  TranslationZOffset=0  TranslationZOffsetUnits=m  TranslationThetaOffset=0  TranslationThetaOffsetUnits=deg  RotationMethod=None  RotationAngleUnits=deg  RotationStandardAxis=+Z  RotationAngle=0.0  RotationArbitraryAxis=[0 0 1]  FollAlignAxisA=+X  BaseAlignAxisA=+Y  FollAlignAxisB=+Y  BaseAlignAxisB=+Z  RotationSequenceAxes=FollowerAxes  RotationSequence=XYX  RotationSequenceAngles=[0 0 0]  RotationSequenceAnglesUnits=deg  RotationMatrix=[1 0 0; 0 1 0; 0 0 1]
  Ground : PMIOPort  Side=Right
  Contact : PMIOPort  Port=2  Side=Left
  connections:
  Earth/RConn1 -- Displacement/LConn1
  Contact/RConn1 -- Earth/LConn1
  Ground/RConn1 -- Transform Launch/LConn1 -- Displacement/RConn1
  Launch Ring/RConn1 -- Launch Insignia/RConn1 -- Transform Launch/RConn1

== system Drone_Simulation/PLANT MODEL/ENVIRONMENT/Sky ==
  Aft Sky : sm_lib/Body Elements/Brick Solid  GraphicAmbientColor=[0.15 0.15 0.15 1.0]  BasedOnType=Density  BrickDimensions=[E E P]  BrickDimensionUnits=m  CenterOfMass=[0 0 0]  CenterOfMassUnits=m  GraphicDiffuseColor=rgbS  Density=rhoS  DensityUnits=kg/m^3  DoExposeReferenceFrame=on  GraphicEmissiveColor=[0.0 0.0 0.0 1.0]  ExportEntireGeometry=off  SerializedFrames=<Frames/>  MarkerShape=Sphere  MarkerSize=10  GraphicType=FromGeometry  InertiaType=CalculateFromGeometry  Mass=1  MassUnits=kg  MomentsOfInertia=[1 1 1]  MomentsOfInertiaUnits=kg*m^2  GraphicOpacity=opS  ProductsOfInertia=[0 0 0]  ProductsOfInertiaUnits=kg*m^2  GraphicShininess=75  GraphicSpecularColor=[0.5 0.5 0.5 1.0]  GraphicVisPropType=SimpleVisualProperties
  Displacement1 : sm_lib/Frames and Transforms/Rigid Transform  TranslationMethod=Cartesian  TranslationStandardOffset=E/2  TranslationLengthUnit=m  TranslationStandardAxis=+Z  TranslationCartesianOffset=[0 -E/2+Z+P E/2+P/2]  TranslationROffset=0  TranslationROffsetUnits=m  TranslationZOffset=0  TranslationZOffsetUnits=m  TranslationThetaOffset=0  TranslationThetaOffsetUnits=deg  RotationMethod=StandardAxis  RotationAngleUnits=deg  RotationStandardAxis=-X  RotationAngle=90  RotationArbitraryAxis=[0 0 1]  FollAlignAxisA=+X  BaseAlignAxisA=+Y  FollAlignAxisB=+Y  BaseAlignAxisB=+Z  RotationSequenceAxes=FollowerAxes  RotationSequence=XYX  RotationSequenceAngles=[0 0 0]  RotationSequenceAnglesUnits=deg  RotationMatrix=[1 0 0; 0 1 0; 0 0 1]
  Displacement6 : sm_lib/Frames and Transforms/Rigid Transform  TranslationMethod=Cartesian  TranslationStandardOffset=E/2  TranslationLengthUnit=m  TranslationStandardAxis=+Z  TranslationCartesianOffset=[E/2-Z-P 0 E/2+P/2]  TranslationROffset=0  TranslationROffsetUnits=m  TranslationZOffset=0  TranslationZOffsetUnits=m  TranslationThetaOffset=0  TranslationThetaOffsetUnits=deg  RotationMethod=StandardAxis  RotationAngleUnits=deg  RotationStandardAxis=-Y  RotationAngle=90  RotationArbitraryAxis=[0 0 1]  FollAlignAxisA=+X  BaseAlignAxisA=+Y  FollAlignAxisB=+Y  BaseAlignAxisB=+Z  RotationSequenceAxes=FollowerAxes  RotationSequence=XYX  RotationSequenceAngles=[0 0 0]  RotationSequenceAnglesUnits=deg  RotationMatrix=[1 0 0; 0 1 0; 0 0 1]
  Left Sky : sm_lib/Body Elements/Brick Solid  GraphicAmbientColor=[0.15 0.15 0.15 1.0]  BasedOnType=Density  BrickDimensions=[E E P]  BrickDimensionUnits=m  CenterOfMass=[0 0 0]  CenterOfMassUnits=m  GraphicDiffuseColor=rgbS  Density=rhoS  DensityUnits=kg/m^3  DoExposeReferenceFrame=on  GraphicEmissiveColor=[0.0 0.0 0.0 1.0]  ExportEntireGeometry=off  SerializedFrames=<Frames/>  MarkerShape=Sphere  MarkerSize=10  GraphicType=FromGeometry  InertiaType=CalculateFromGeometry  Mass=1  MassUnits=kg  MomentsOfInertia=[1 1 1]  MomentsOfInertiaUnits=kg*m^2  GraphicOpacity=opS  ProductsOfInertia=[0 0 0]  ProductsOfInertiaUnits=kg*m^2  GraphicShininess=75  GraphicSpecularColor=[0.5 0.5 0.5 1.0]  GraphicVisPropType=SimpleVisualProperties
  Sky : PMIOPort  Side=Right
  connections:
  Displacement6/LConn1 -- Left Sky/RConn1
  Displacement1/LConn1 -- Aft Sky/RConn1
  Sky/RConn1 -- Displacement1/RConn1 -- Displacement6/RConn1
